simulink library "SEA_library_controllers"  (Simulink 8.6)
settings: Solver=ode45  StartTime=0.0  StopTime=10.0  RelTol=1e-3
values from neighbouring files (symbols this model uses):
  N = this.jointModel.n    [dataSheetGenerator.m]
undefined symbols (not defined in the file or in its folder): Cc, DiscIntNeverNeededParam, jointObj, K_lqr, Kd, kest, Ki, Kp
undefined symbols (not defined in the file): joint_DOB, My_joint, W2k_output_fixed_coulomb
libraries: cstblocks x6, SEA_library_observers x1
settings Model: Creator=wesley  LastModifiedBy=wesley

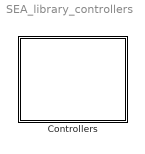
== system SEA_library_controllers ==
  Controllers : Subsystem

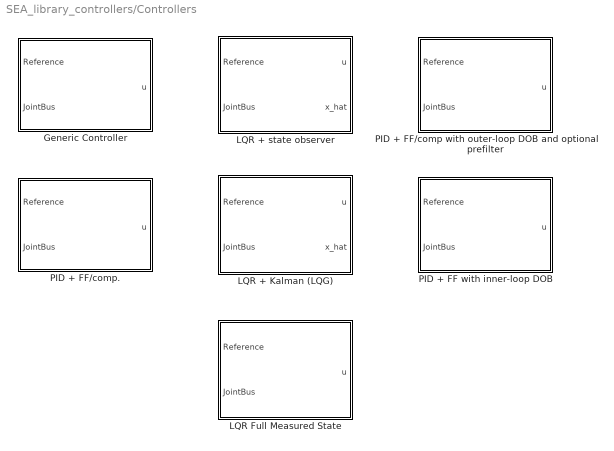
== system SEA_library_controllers/Controllers ==
  Generic Controller : Subsystem  mask{jointObj=My_joint}
      mask prompts: jointObj "Joint Object"
      mask init:
      | % Get linear dynamics matrices
      | [A, B, C, I, D, K] = jointObj.getDynamicsMatrices();
  LQR + Kalman (LQG) : Subsystem  mask{jointObj=My_joint, outputIdx=3, Q=diag([0 0 1000 0 0 0]), R=5e-6, var_u=0.12^2, var_y=1.8e-10}
      mask prompts: jointObj "Joint Object (fixed output model)"; outputIdx "Measured output"; Q "State weighing matrix Q"; R "Input weighing matrix R"; var_u "Input noise variance"; var_y "Measurement noise variance"
      mask init:
      | % Get linear dynamics matrices
      | [A, B, C, D] = jointObj.getDynamicsMatrices();
      | 
      | % Parameters
      | N_outputs       = size(C,1);
      | 
      | % Get LQR gain and Kalman observer
      | [K_lqr, N]  	= getLQR(jointObj, outputIdx, Q, R);
      | [kest, L, Cc]	= getKalman(jointObj, outputIdx, var_u, var_y);
      | 
      | % Indexes of output states
      | kest_stateIdx   = kest.OutputGroup.StateEstimate;
      | 
      | % Discretize using Tustin transform
      | kest_tust       = c2d(kest, jointObj.Ts, 'tustin');
  LQR + state observer : Subsystem  mask{jointObj=My_joint, outputIdx=3, Q=diag([0 0 1000 0 0 0]), R=5e-6, place_gain=4}
      mask prompts: jointObj "Joint Object"; outputIdx "Measured output"; Q "State weighing matrix Q"; R "Input weighing matrix R"; place_gain "Pole placement gain"
      mask init:
      | % Get linear dynamics matrices
      | [A, B, C, D] = jointObj.getDynamicsMatrices();
      | 
      | % Parameters
      | N_outputs = size(C,1);
      | 
      | % Get LQR gain and state observer
      | [K_lqr, N]          = getLQR(jointObj, outputIdx, Q, R);
      | [sys_hat, L, Cc]	= getObserver(jointObj, outputIdx, place_gain, Q, R);
      | 
      | % Discretize using Tustin transform
      | sys_hat_tust = c2d(sys_hat, jointObj.Ts, 'tustin');
  LQR Full Measured State : Subsystem  mask{jointObj=My_joint, outputIdx=3, Q=diag([0 0 1000 0 0 0]), R=5e-6}
      mask prompts: jointObj "Joint Object"; outputIdx "Measured output"; Q "State weighing matrix Q"; R "Input weighing matrix R"
      mask init:
      | % Get linear dynamics matrices
      | [A, B, C, D] = jointObj.getDynamicsMatrices();
      | 
      | % Get LQR gain and premultiplication matrix N
      | [K_lqr, N]          = getLQR(jointObj, outputIdx, Q, R);
      | 
      | % Get selector to obtain full state from outputs y
      | % This makes use of the fact that the first 6 outputs are the states
      | outputToStates      = C(1:6,:)';
  PID + FF with inner-loop DOB : Subsystem  mask{jointObj=joint_DOB, Kp=Kp, Ki=Ki, Kd=Kd, N=2*pi*200, ff_comp_switch=Feed-forward, f_c=100, measIdx=[7], doPlot=off}
      mask prompts: jointObj "Joint Object"; Kp "Proportional gain Kp"; Ki "Integral gain Ki"; Kd "Derivative gain Kd"; N "Filter coefficient N"; ff_comp_switch "Spring force rejection"; f_c "DOB cut-off frequency [Hz]"; measIdx "Measurement index"; doPlot "Do plot"
      mask init:
      | % Get linear dynamics matrices
      | [A, B, C, D, I, R, K] = jointObj.getDynamicsMatrices();
      mask TypeOptions ff_comp_switch: Compensation | Feed-forward | Off
      mask DialogControl Container3 Prompt: Controller
      mask DialogControl ParameterGroupVar Prompt: DOB parameters
  PID + FF/comp with outer-loop DOB and optional prefilter : Subsystem  mask{jointObj=W2k_output_fixed_coulomb, Kp=0.35, Ki=0, Kd=(2*(jointObj.I_m + jointObj.I_g)*sqrt((jointObj.k_b * jointObj.k_t * 0.35 * jointObj.n + jointObj.k_b)/(jointObj.I_m + jointObj.I_g))*1.2 - (jointObj.d_m + jointObj.d_g + jointObj.d_gb)) / (jointObj.k_b * jointObj.k_t * jointObj.n), N=2*pi*200, ff_comp_switch=Feed-forward, DOB_enable_switch=Off, premult_enable_switch=On, loadData=off, modelFname=DOB_results.mat, f_c_FF=50, f_c_DOB=100}
      mask prompts: jointObj "Joint Object"; Kp "Proportional gain Kp"; Ki "Integral gain Ki"; Kd "Derivative gain Kd"; N "Derivative filter coefficient N"; ff_comp_switch "Spring force rejection"; DOB_enable_switch "DOB"; premult_enable_switch "Premultiplication"; loadData "Load model/filters from file (see getLinearDOB_fromData)"; modelFname "Model/filters file (.mat)"; f_c_FF "Premultiplication (model inversion) cutoff frequency [Hz]"; f_c_DOB "DOB cutoff frequency [Hz]"
      mask init:
      | % Calculate the approximated closed-loop transfer function Pc and
      | % filters Q_* etc.
      | % This is the standalone code, that does not require measurement data
      | % from a simulink model to design the model.
      | % However, it uses a linear state-space model to estimate the transfer
      | % function of the plant, thus the results are fundamentally different from
      | % the experimental version.
      | 
      | % Get linear dynamics matrices
      | [A, B, C, I, D, K] = jointObj.getDynamicsMatrices();
      | 
      | % Default values (off)
      | Q_td    = tf(0);
      | PQ_td	= tf(0);
      | PQ_ff	= tf(0);
      | 
      | % Check if DOB is enabled
      | if (DOB_enable_switch == 2)
      |     % If filename is given, assume the model and filters can be found in there
      |     if (loadData)
      |         if (isempty(modelFname))
      |             error('Error: Model/filters data file not found!');
      |         else
      |             % Load file and exit
      |             load(modelFname);
      |         end
      |     else
      |         %% If no filename is given with model&filters from experimental identifica-
      |         % tion, do a linear simulation to obtain their approximate values (this
      |         % will significantly influence the results)
      | 
      |         [Pc, Q_td, Q_ff, PQ_td, PQ_ff] = design_DOB_controller( jointObj, ...
      |                                                                 Kp, Ki, Kd, N, 'parallel', ...
      |                                                                 7, ... % Torque output
      |                                                                 ff_comp_switch, ...
      |                                                                 f_c_FF, f_c_DOB             );
      |     end
      | else
      |     % If the DOB is disabled, make sure the prefilter is also disabled
      |     premult_enable_switch = 1;
      | end
      | 
      | % Discretize using Tustin transform
      | Q_td_tust	= c2d(Q_td, jointObj.Ts, 'tustin');
      | PQ_td_tust	= c2d(PQ_td, jointObj.Ts, 'tustin');
      | PQ_ff_tust  = c2d(PQ_ff, jointObj.Ts, 'tustin');
      mask TypeOptions ff_comp_switch: Compensation | Feed-forward | Off
      mask TypeOptions DOB_enable_switch: Off | On
      mask Callback DOB_enable_switch:
      | % Toggle all DOB fields
      | fields = {  'premult_enable_switch', ...
      |             'loadData', ...
      |             'modelFname', ...
      |             'id_Np', ...
      |             'id_Nz', ...
      |             'f_c_FF', ...
      |             'f_c_DOB', ...
      |          };
      | toggleMaskFields(gcbh, 'DOB_enable_switch', fields, 'on');
      | 
      | % File load or model generation
      | if (strcmpi(get(gcbh, 'DOB_enable_switch'), 'on'))
      |     toggleMaskFields(gcbh, 'loadData', 'modelFname', 'on');
      |     toggleMaskFields(gcbh, 'loadData', {'f_c_FF', 'f_c_DOB'}, 'off');
      | end
      mask TypeOptions premult_enable_switch: Off | On
      mask Callback loadData:
      | if (strcmpi(get(gcbh, 'DOB_enable_switch'), 'on'))
      |     toggleMaskFields(gcbh, 'loadData', 'modelFname', 'on');
      |     toggleMaskFields(gcbh, 'loadData', {'button_build_DOB', 'f_c', 'id_Np', 'id_Nz', 'f_c_FF', 'f_c_DOB'}, 'off');
      | end
      mask DialogControl Container2 Prompt: Controller
      mask DialogControl DOB_container Prompt: DOB and premultiplication
      mask DialogControl DOB_analytical_container Prompt: Analytical DOB
  PID + FF/comp. : Subsystem  mask{jointObj=My_joint, Kp=0.35, Ki=0, Kd=(2*(jointObj.I_m + jointObj.I_g)*sqrt((jointObj.k_b * jointObj.k_t * 0.35 * jointObj.n + jointObj.k_b)/(jointObj.I_m + jointObj.I_g))*1.2 - (jointObj.d_m + jointObj.d_g + jointObj.d_gb)) / (jointObj.k_b * jointObj.k_t * jointObj.n), N=2*pi*200, ff_comp_switch=Feed-forward}
      mask prompts: jointObj "Joint Object"; Kp "Proportional gain Kp"; Ki "Integral gain Ki"; Kd "Derivative gain Kd"; N "Filter coefficient N"; ff_comp_switch "Spring force rejection"
      mask init:
      | % Get linear dynamics matrices
      | [A, B, C, D, I, R, K] = jointObj.getDynamicsMatrices();
      mask TypeOptions ff_comp_switch: Compensation | Feed-forward | Off

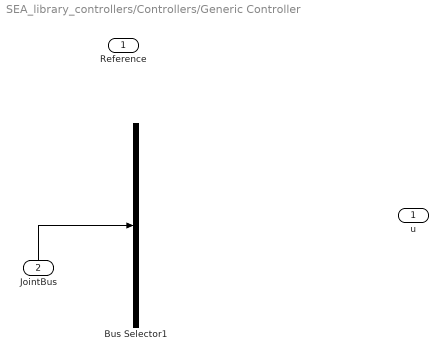
== system SEA_library_controllers/Controllers/Generic Controller ==
  Reference : Inport
  JointBus : Inport  Port=2
  Bus Selector1 : BusSelector  OutputSignals=GearPos,LinkPos,Torque
  u : Outport
  wires:
  JointBus/1 -> Bus Selector1/1

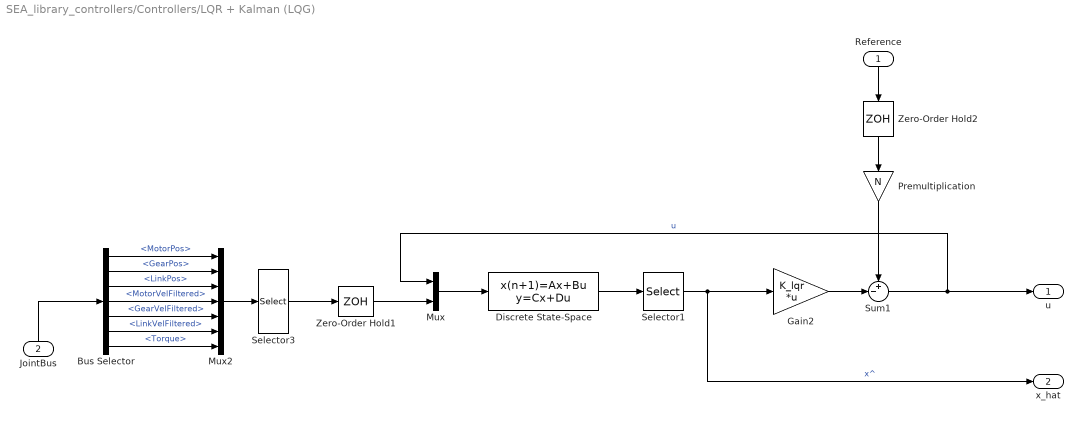
== system SEA_library_controllers/Controllers/LQR + Kalman (LQG) ==
  Reference : Inport
  JointBus : Inport  Port=2
  Bus Selector : BusSelector  OutputSignals=MotorPos,GearPos,LinkPos,MotorVelFiltered,GearVelFiltered,LinkVelFiltered,Torque
  Discrete State-Space : DiscreteStateSpace  A=kest_tust.a  B=kest_tust.b  C=kest_tust.c  D=kest_tust.d  SampleTime=jointObj.Ts
  Gain2 : Gain  Gain=K_lqr  Multiplication=Matrix(K*u)
  Mux : Mux  Inputs=2
  Mux2 : Mux  Inputs=7
  Premultiplication : Gain  Gain=N
  Selector1 : Selector  InputPortWidth=size(kest.c,1)  IndexOptions=Index vector (dialog)  Indices=kest_stateIdx  OutputSizes=1
  Selector3 : Selector  InputPortWidth=N_outputs  IndexOptions=Index vector (dialog)  Indices=outputIdx  OutputSizes=1
  Sum1 : Sum  Inputs=+-|
  Zero-Order Hold1 : ZeroOrderHold  SampleTime=jointObj.Ts
  Zero-Order Hold2 : ZeroOrderHold  SampleTime=jointObj.Ts
  u : Outport
  x_hat : Outport  Port=2
  wires:
  Discrete State-Space/1 -> Selector1/1
  Mux/1 -> Discrete State-Space/1
  Gain2/1 -> Sum1/2
  Premultiplication/1 -> Sum1/1
  Reference/1 -> Zero-Order Hold2/1
  Sum1/1 -> u/1, Mux/1  "u"
  Bus Selector/7 -> Mux2/7  "<Torque>"
  Mux2/1 -> Selector3/1
  Bus Selector/1 -> Mux2/1  "<MotorPos>"
  Bus Selector/5 -> Mux2/5  "<GearVelFiltered>"
  Bus Selector/3 -> Mux2/3  "<LinkPos>"
  Bus Selector/6 -> Mux2/6  "<LinkVelFiltered>"
  Bus Selector/2 -> Mux2/2  "<GearPos>"
  Bus Selector/4 -> Mux2/4  "<MotorVelFiltered>"
  JointBus/1 -> Bus Selector/1
  Selector3/1 -> Zero-Order Hold1/1
  Selector1/1 -> x_hat/1, Gain2/1  "x^"
  Zero-Order Hold1/1 -> Mux/2
  Zero-Order Hold2/1 -> Premultiplication/1

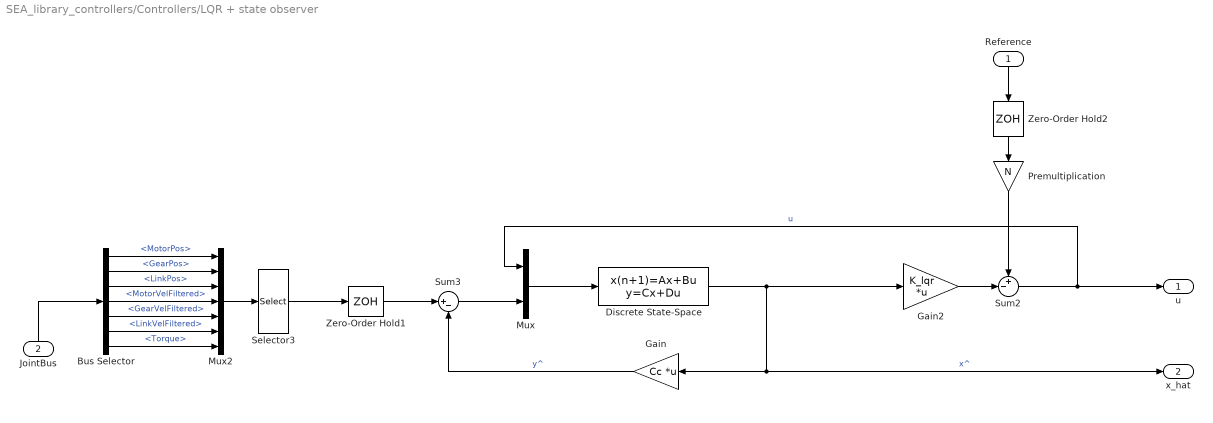
== system SEA_library_controllers/Controllers/LQR + state observer ==
  Reference : Inport
  JointBus : Inport  Port=2
  Bus Selector : BusSelector  OutputSignals=MotorPos,GearPos,LinkPos,MotorVelFiltered,GearVelFiltered,LinkVelFiltered,Torque
  Discrete State-Space : DiscreteStateSpace  A=sys_hat_tust.a  B=sys_hat_tust.b  C=sys_hat_tust.c  D=sys_hat_tust.d  SampleTime=jointObj.Ts
  Gain : Gain  Gain=Cc  Multiplication=Matrix(K*u)
  Gain2 : Gain  Gain=K_lqr  Multiplication=Matrix(K*u)
  Mux : Mux  Inputs=2
  Mux2 : Mux  Inputs=7
  Premultiplication : Gain  Gain=N
  Selector3 : Selector  InputPortWidth=N_outputs  IndexOptions=Index vector (dialog)  Indices=outputIdx  OutputSizes=1
  Sum2 : Sum  Inputs=+-|
  Sum3 : Sum  Inputs=|+-
  Zero-Order Hold1 : ZeroOrderHold  SampleTime=jointObj.Ts
  Zero-Order Hold2 : ZeroOrderHold  SampleTime=jointObj.Ts
  u : Outport
  x_hat : Outport  Port=2
  wires:
  Zero-Order Hold2/1 -> Premultiplication/1
  Zero-Order Hold1/1 -> Sum3/1
  Reference/1 -> Zero-Order Hold2/1
  Sum2/1 -> u/1, Mux/1  "u"
  Premultiplication/1 -> Sum2/1
  Gain2/1 -> Sum2/2
  Mux/1 -> Discrete State-Space/1
  Selector3/1 -> Zero-Order Hold1/1
  Sum3/1 -> Mux/2
  Gain/1 -> Sum3/2  "y^"
  JointBus/1 -> Bus Selector/1
  Bus Selector/4 -> Mux2/4  "<MotorVelFiltered>"
  Bus Selector/2 -> Mux2/2  "<GearPos>"
  Bus Selector/6 -> Mux2/6  "<LinkVelFiltered>"
  Bus Selector/3 -> Mux2/3  "<LinkPos>"
  Bus Selector/5 -> Mux2/5  "<GearVelFiltered>"
  Bus Selector/1 -> Mux2/1  "<MotorPos>"
  Mux2/1 -> Selector3/1
  Discrete State-Space/1 -> x_hat/1, Gain/1, Gain2/1  "x^"
  Bus Selector/7 -> Mux2/7  "<Torque>"

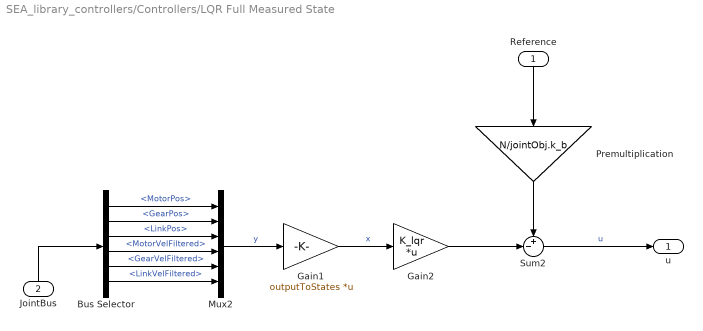
== system SEA_library_controllers/Controllers/LQR Full Measured State ==
  Reference : Inport
  JointBus : Inport  Port=2
  Bus Selector : BusSelector  OutputSignals=MotorPos,GearPos,LinkPos,MotorVelFiltered,GearVelFiltered,LinkVelFiltered
  Gain1 : Gain  Gain=outputToStates  Multiplication=Matrix(K*u)
  Gain2 : Gain  Gain=K_lqr  Multiplication=Matrix(K*u)
  Mux2 : Mux  Inputs=6
  Premultiplication : Gain  Gain=N/jointObj.k_b
  Sum2 : Sum  Inputs=+-|
  u : Outport
  wires:
  Gain1/1 -> Gain2/1  "x"
  Bus Selector/1 -> Mux2/1  "<MotorPos>"
  Bus Selector/5 -> Mux2/5  "<GearVelFiltered>"
  Bus Selector/3 -> Mux2/3  "<LinkPos>"
  Bus Selector/6 -> Mux2/6  "<LinkVelFiltered>"
  Bus Selector/2 -> Mux2/2  "<GearPos>"
  Bus Selector/4 -> Mux2/4  "<MotorVelFiltered>"
  JointBus/1 -> Bus Selector/1
  Gain2/1 -> Sum2/2
  Premultiplication/1 -> Sum2/1
  Sum2/1 -> u/1  "u"
  Reference/1 -> Premultiplication/1
  Mux2/1 -> Gain1/1  "y"

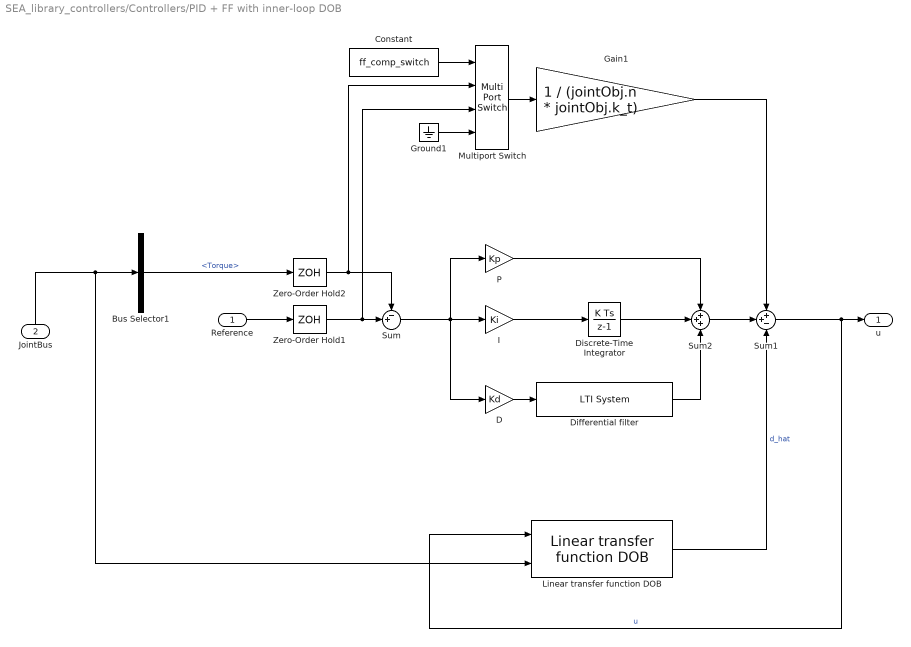
== system SEA_library_controllers/Controllers/PID + FF with inner-loop DOB ==
  Reference : Inport
  JointBus : Inport  Port=2
  Bus Selector1 : BusSelector  OutputSignals=Torque
  Constant : Constant  Value=ff_comp_switch
  D : Gain  Gain=Kd
  Differential filter : cstblocks/LTI System  sys=c2d(tf([N 0], [1, N]), jointObj.Ts, 'tustin')  IC=[]
  Discrete-Time Integrator : DiscreteIntegrator  SampleTime=-1  ICPrevOutput=DiscIntNeverNeededParam  ICPrevScaledInput=DiscIntNeverNeededParam
  Gain1 : Gain  Gain=1 / (jointObj.n * jointObj.k_t)
  Ground1 : Ground
  I : Gain  Gain=Ki
  Linear transfer function DOB : SEA_library_observers/Observers/Linear transfer function DOB  loadData=off  modelFname=DOB_inner_results.mat  jointObj=jointObj  f_c=f_c  measIdx=measIdx  doPlot=off
  Multiport Switch : MultiPortSwitch
  P : Gain  Gain=Kp
  Sum : Sum  Inputs=-+|
  Sum1 : Sum  Inputs=++-
  Sum2 : Sum  Inputs=+++
  Zero-Order Hold1 : ZeroOrderHold  SampleTime=jointObj.Ts
  Zero-Order Hold2 : ZeroOrderHold  SampleTime=jointObj.Ts
  u : Outport
  wires:
  Zero-Order Hold2/1 -> Sum/1, Multiport Switch/2
  Zero-Order Hold1/1 -> Sum/2, Multiport Switch/3
  Ground1/1 -> Multiport Switch/4
  Multiport Switch/1 -> Gain1/1
  Constant/1 -> Multiport Switch/1
  Gain1/1 -> Sum1/1
  Reference/1 -> Zero-Order Hold1/1
  Sum1/1 -> Linear transfer function DOB/1, u/1  "u"
  Bus Selector1/1 -> Zero-Order Hold2/1  "<Torque>"
  JointBus/1 -> Linear transfer function DOB/2, Bus Selector1/1
  Linear transfer function DOB/1 -> Sum1/3  "d_hat"
  D/1 -> Differential filter/1
  I/1 -> Discrete-Time Integrator/1
  Discrete-Time Integrator/1 -> Sum2/2
  P/1 -> Sum2/1
  Differential filter/1 -> Sum2/3
  Sum2/1 -> Sum1/2
  Sum/1 -> D/1, I/1, P/1

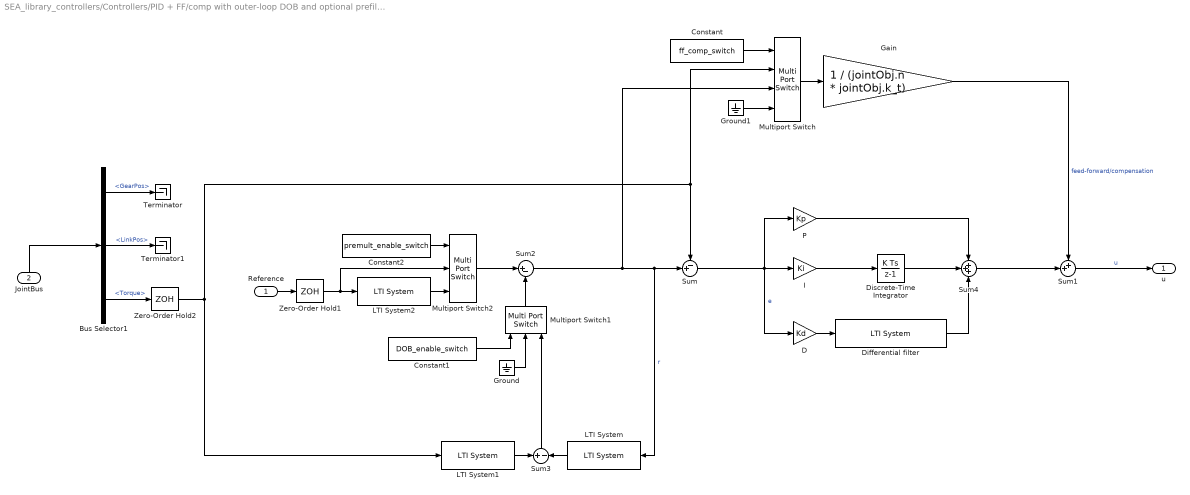
== system SEA_library_controllers/Controllers/PID + FF/comp with outer-loop DOB and optional prefilter ==
  Reference : Inport
  JointBus : Inport  Port=2
  Bus Selector1 : BusSelector  OutputSignals=GearPos,LinkPos,Torque
  Constant : Constant  Value=ff_comp_switch
  Constant1 : Constant  Value=DOB_enable_switch
  Constant2 : Constant  Value=premult_enable_switch
  D : Gain  Gain=Kd
  Differential filter : cstblocks/LTI System  sys=c2d(tf([N 0], [1, N]), jointObj.Ts, 'tustin')  IC=[]
  Discrete-Time Integrator : DiscreteIntegrator  SampleTime=-1  ICPrevOutput=DiscIntNeverNeededParam  ICPrevScaledInput=DiscIntNeverNeededParam
  Gain : Gain  Gain=1 / (jointObj.n * jointObj.k_t)
  Ground : Ground
  Ground1 : Ground
  I : Gain  Gain=Ki
  LTI System : cstblocks/LTI System  sys=Q_td_tust  IC=[]
  LTI System1 : cstblocks/LTI System  sys=PQ_td_tust  IC=[]
  LTI System2 : cstblocks/LTI System  sys=PQ_ff_tust  IC=[]
  Multiport Switch : MultiPortSwitch
  Multiport Switch1 : MultiPortSwitch  Inputs=2
  Multiport Switch2 : MultiPortSwitch  Inputs=2
  P : Gain  Gain=Kp
  Sum : Sum  Inputs=-+|
  Sum1 : Sum  Inputs=++|
  Sum2 : Sum  Inputs=|+-
  Sum3 : Sum  Inputs=+|-
  Sum4 : Sum  Inputs=+++
  Terminator : Terminator
  Terminator1 : Terminator
  Zero-Order Hold1 : ZeroOrderHold  SampleTime=jointObj.Ts
  Zero-Order Hold2 : ZeroOrderHold  SampleTime=jointObj.Ts
  u : Outport
  wires:
  Multiport Switch2/1 -> Sum2/1
  Zero-Order Hold1/1 -> LTI System2/1, Multiport Switch2/2
  Zero-Order Hold2/1 -> LTI System1/1, Multiport Switch/2, Sum/1
  Reference/1 -> Zero-Order Hold1/1
  Ground1/1 -> Multiport Switch/4
  Bus Selector1/2 -> Terminator1/1  "<LinkPos>"
  Bus Selector1/1 -> Terminator/1  "<GearPos>"
  JointBus/1 -> Bus Selector1/1
  Bus Selector1/3 -> Zero-Order Hold2/1  "<Torque>"
  Sum1/1 -> u/1  "u"
  Gain/1 -> Sum1/1  "feed-forward/compensation"
  Sum2/1 -> LTI System/1, Sum/2, Multiport Switch/3  "r"
  LTI System1/1 -> Sum3/1
  LTI System/1 -> Sum3/2
  Sum3/1 -> Multiport Switch1/3
  LTI System2/1 -> Multiport Switch2/3
  Multiport Switch/1 -> Gain/1
  Constant/1 -> Multiport Switch/1
  Multiport Switch1/1 -> Sum2/2
  Ground/1 -> Multiport Switch1/2
  Constant1/1 -> Multiport Switch1/1
  Constant2/1 -> Multiport Switch2/1
  D/1 -> Differential filter/1
  I/1 -> Discrete-Time Integrator/1
  Discrete-Time Integrator/1 -> Sum4/2
  P/1 -> Sum4/1
  Differential filter/1 -> Sum4/3
  Sum4/1 -> Sum1/2
  Sum/1 -> D/1, I/1, P/1  "e"

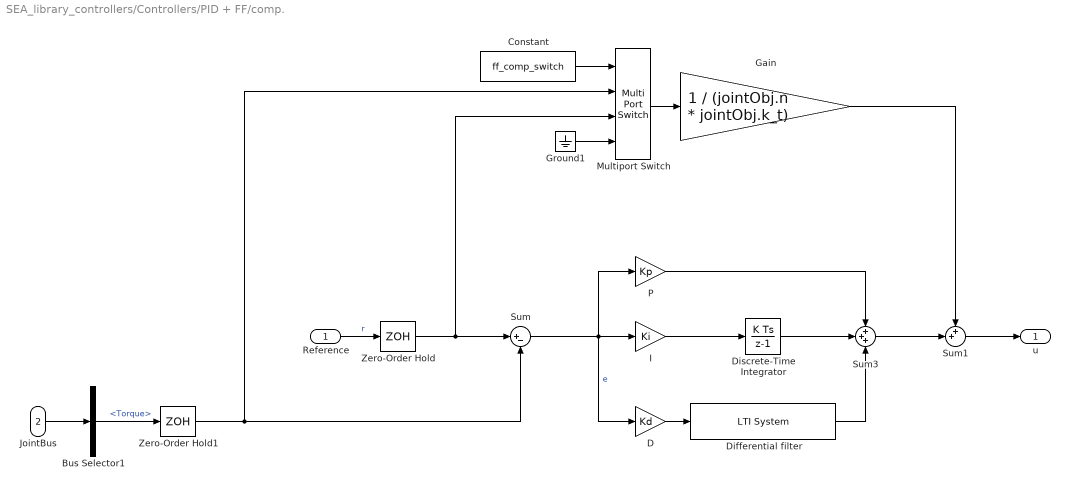
== system SEA_library_controllers/Controllers/PID + FF/comp. ==
  Reference : Inport
  JointBus : Inport  Port=2
  Bus Selector1 : BusSelector  OutputSignals=Torque
  Constant : Constant  Value=ff_comp_switch
  D : Gain  Gain=Kd
  Differential filter : cstblocks/LTI System  sys=c2d(tf([N 0], [1, N]), jointObj.Ts, 'tustin')  IC=[]
  Discrete-Time Integrator : DiscreteIntegrator  SampleTime=-1  ICPrevOutput=DiscIntNeverNeededParam  ICPrevScaledInput=DiscIntNeverNeededParam
  Gain : Gain  Gain=1 / (jointObj.n * jointObj.k_t)
  Ground1 : Ground
  I : Gain  Gain=Ki
  Multiport Switch : MultiPortSwitch
  P : Gain  Gain=Kp
  Sum : Sum  Inputs=|+-
  Sum1 : Sum  Inputs=++|
  Sum3 : Sum  Inputs=+++
  Zero-Order Hold : ZeroOrderHold  SampleTime=jointObj.Ts
  Zero-Order Hold1 : ZeroOrderHold  SampleTime=jointObj.Ts
  u : Outport
  wires:
  Zero-Order Hold1/1 -> Sum/2, Multiport Switch/2
  Zero-Order Hold/1 -> Multiport Switch/3, Sum/1
  Sum/1 -> P/1, I/1, D/1  "e"
  Sum3/1 -> Sum1/2
  Differential filter/1 -> Sum3/3
  P/1 -> Sum3/1
  Discrete-Time Integrator/1 -> Sum3/2
  I/1 -> Discrete-Time Integrator/1
  D/1 -> Differential filter/1
  Sum1/1 -> u/1
  JointBus/1 -> Bus Selector1/1
  Ground1/1 -> Multiport Switch/4
  Bus Selector1/1 -> Zero-Order Hold1/1  "<Torque>"
  Reference/1 -> Zero-Order Hold/1  "r"
  Multiport Switch/1 -> Gain/1
  Constant/1 -> Multiport Switch/1
  Gain/1 -> Sum1/1
